simulink model "InvertedPendulum_Simulink2017aLQR"  (R2022a)
settings: Solver=ode4  StartTime=0.0  StopTime=SIM_TIME  FixedStep=STEP_SIZE  RelTol=1e-3
undefined symbols (not defined in the file or in its folder): b, c, g, I, K, Ke, Kt, l, m, M, R, r, theta0, theta_dot0, Ts, x0, x_dot0
settings Model: Creator=roga  LastModifiedBy=farfar
settings SolverCC: AlgebraicLoopSolver=TrustRegion
settings DataIOCC: ExternalInput=[0 0]  InitialState=[]  ReturnWorkspaceOutputs=off
settings OptimizationCC: DefaultParameterBehavior=Inlined  BufferReuse=off
settings DebuggingCC: AlgebraicLoopMsg=none  UnconnectedInputMsg=warning  UnconnectedOutputMsg=warning  UnconnectedLineMsg=warning  InitInArrayFormatMsg=none  SFMachineParentedDataDiag=warning  ArithmeticOperatorsInVariantConditions=warning
settings SFSimCC: CustomCodeUndefinedFunction=UseInterfaceOnly
settings CodeAppCC: StateflowObjectComments=on

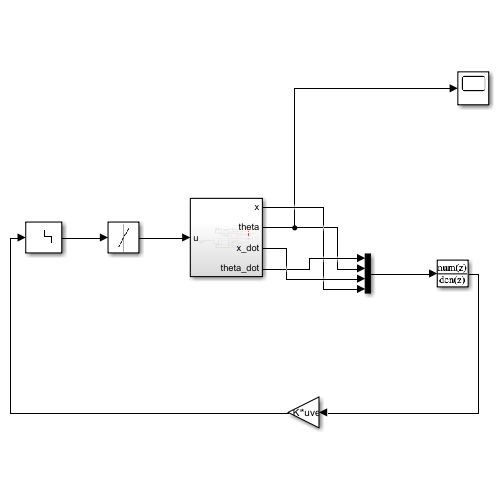
[thumbnail: Simulink's stored preview of the top-level diagram]
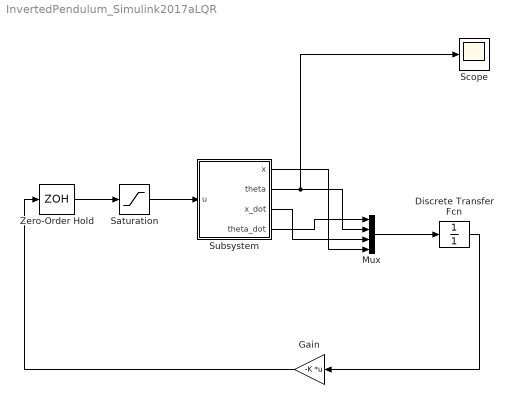
== system InvertedPendulum_Simulink2017aLQR ==
  Discrete Transfer Fcn : DiscreteTransferFcn  Denominator=[1]  SampleTime=Ts
  Gain : Gain  Gain=-K  Multiplication=Matrix(K*u) (u vector)
  Mux : Mux
  Saturation : Saturate  UpperLimit=12  LowerLimit=-12
  Scope : Scope
  Subsystem : Subsystem
  Zero-Order Hold : ZeroOrderHold  SampleTime=Ts
  wires:
  Subsystem/4(theta_dot) -> Mux/1
  Subsystem/2(theta) -> Scope/1, Mux/2
  Subsystem/3(x_dot) -> Mux/3
  Subsystem/1(x) -> Mux/4
  Mux/1 -> Discrete Transfer Fcn/1
  Discrete Transfer Fcn/1 -> Gain/1
  Zero-Order Hold/1 -> Saturation/1
  Gain/1 -> Zero-Order Hold/1
  Saturation/1 -> Subsystem/1(u)

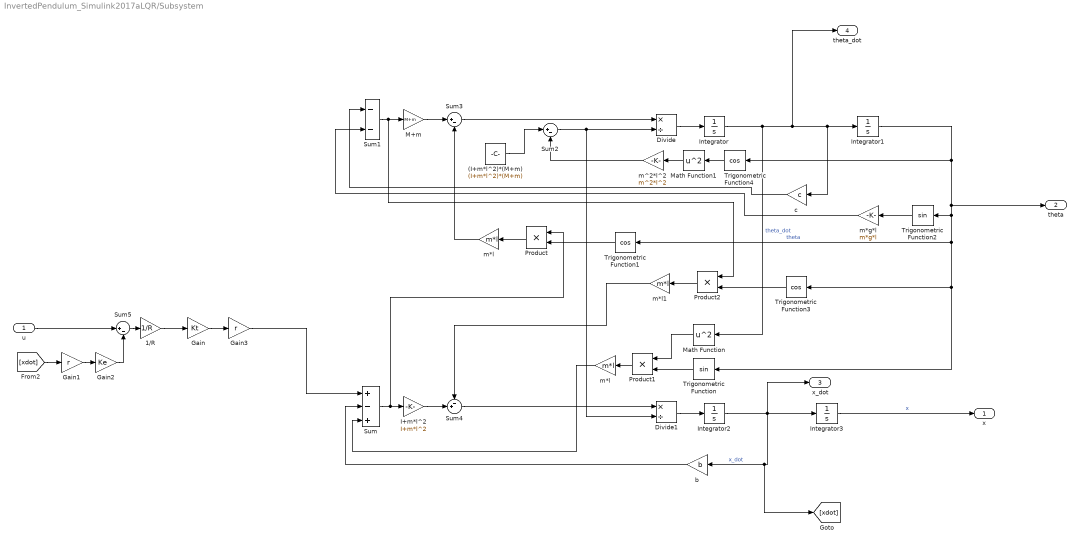
== system InvertedPendulum_Simulink2017aLQR/Subsystem ==
  u : Inport
  (I+m*l^2)*(M+m) : Constant  Value=(I+m*l^2)*(M+m)
  1/R : Gain  Gain=1/R
  Divide : Product  Inputs=*/
  Divide1 : Product  Inputs=*/
  Gain : Gain  Gain=Kt
  Gain1 : Gain  Gain=r
  Gain2 : Gain  Gain=Ke
  Gain3 : Gain  Gain=r
  I+m*l^2 : Gain  Gain=I+m*l^2
  Integrator : Integrator  Priority=1  InitialCondition=theta_dot0  ContinuousStateAttributes='pendulum.angular.velocity'
  Integrator1 : Integrator  Priority=2  InitialCondition=theta0  UpperSaturationLimit=pi  LowerSaturationLimit=-pi  ContinuousStateAttributes='pendulum.angular.position'
  Integrator2 : Integrator  Priority=3  InitialCondition=x_dot0  ContinuousStateAttributes='trolley.horizontal.velocity'
  Integrator3 : Integrator  Priority=4  InitialCondition=x0  ContinuousStateAttributes='trolley.horizontal.position'
  M+m : Gain  Gain=M+m
  Math Function : Math  Operator=square  SignedPower=on
  Math Function1 : Math  Operator=square  SignedPower=on
  Product : Product
  Product1 : Product
  Product2 : Product
  Sum : Sum  Inputs=+-+
  Sum1 : Sum  Inputs=--
  Sum2 : Sum  Inputs=|+-
  Sum3 : Sum  Inputs=|+-
  Sum4 : Sum  Inputs=-+|
  Sum5 : Sum  Inputs=|+-
  Trigonometric Function : Trigonometry
  Trigonometric Function1 : Trigonometry  Operator=cos
  Trigonometric Function2 : Trigonometry
  Trigonometric Function3 : Trigonometry  Operator=cos
  Trigonometric Function4 : Trigonometry  Operator=cos
  b : Gain  Gain=b
  c : Gain  Gain=c
  m*g*l : Gain  Gain=m*g*l
  m*l : Gain  Gain=m*l
  "m*l " : Gain  Gain=m*l
  m*l1 : Gain  Gain=m*l
  m^2*l^2 : Gain  Gain=m^2*l^2
  x : Outport
  theta : Outport  Port=2
  x_dot : Outport  Port=3
  theta_dot : Outport  Port=4
  wires:
  Integrator/1 -> Math Function/1, theta_dot/1, c/1, Integrator1/1  "theta_dot"
  m*l/1 -> Sum3/2
  (I+m*l^2)*(M+m)/1 -> Sum2/1
  Sum4/1 -> Divide1/1
  Gain1/1 -> Gain2/1
  Math Function1/1 -> m^2*l^2/1
  Sum3/1 -> Divide/1
  Sum/1 -> Product/1, I+m*l^2/1
  Integrator2/1 -> x_dot/1, [xdot], b/1, Integrator3/1  "x_dot"
  Trigonometric Function4/1 -> Math Function1/1
  Trigonometric Function1/1 -> Product/2
  1/R/1 -> Gain/1
  Trigonometric Function/1 -> Product1/2
  Sum2/1 -> Divide1/2, Divide/2
  m*g*l/1 -> Sum1/2
  Trigonometric Function3/1 -> Product2/2
  Product2/1 -> m*l1/1
  Sum1/1 -> Product2/1, M+m/1
  m^2*l^2/1 -> Sum2/2
  M+m/1 -> Sum3/1
  Gain2/1 -> Sum5/2
  Gain3/1 -> Sum/1
  Integrator3/1 -> x/1  "x"
  Integrator1/1 -> Trigonometric Function4/1, theta/1, Trigonometric Function2/1, Trigonometric Function1/1, Trigonometric Function3/1, Trigonometric Function/1  "theta"
  c/1 -> Sum1/1
  I+m*l^2/1 -> Sum4/2
  Math Function/1 -> Product1/1
  "m*l "/1 -> Sum/3
  m*l1/1 -> Sum4/1
  Divide/1 -> Integrator/1
  [xdot] -> Gain1/1
  Trigonometric Function2/1 -> m*g*l/1
  b/1 -> Sum/2
  Product/1 -> m*l/1
  u/1 -> Sum5/1
  Divide1/1 -> Integrator2/1
  Product1/1 -> "m*l "/1
  Sum5/1 -> 1/R/1
  Gain/1 -> Gain3/1
